simulink model "Regler_08"  (R2014b)
settings: Solver=ode45  StartTime=0.0  StopTime=10.0  RelTol=1e-3
values from neighbouring files (symbols this model uses):
  parInit =     [parameter_08.mat]
  parSys =     [parameter_08.mat]
settings Model: CovSFcnEnable=on  Creator=cds-lue-1  LastModifiedBy=cds-lue-1
settings DebuggingCC: SolverPrmCheckMsg=none  FrameProcessingCompatibilityMsg=error

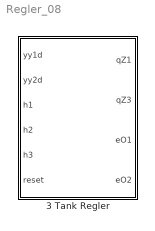
== system Regler_08 ==
  3 Tank Regler : MATLAB Function  TreatAsAtomicUnit=on
      settings: PermitHierarchicalResolution=ParametersOnly

== matlab function Regler_08/3 Tank Regler ==
  settings: updateMethod=DISCRETE  sampleTime=parSys.Ta
  data: qZ1 output; qZ3 output; yy1d input; yy2d input; h1 input; h2 input; h3 input; reset input; parSys parameter; parInit parameter; eO1 output; eO2 output
function [qZ1,qZ3,eO1,eO2]  = fcn(yy1d, yy2d, h1, h2, h3, reset, parSys, parInit)

persistent e1
persistent e2

if isempty(e1)
    e1 = 0;
end

if isempty(e2)
    e2 = 0;
end

if reset
    e1 = 0;
    e2 = 0;
end
    

Atank = parSys.Atank;
rho = parSys.rho;
eta = parSys.eta;
g = parSys.g;
alphaA1 = parSys.alphaA1;
DA1 = parSys.DA1;
alphaA2 = parSys.alphaA2;
A2 = parSys.A2;
alphaA3 = parSys.alphaA3;
DA3 = parSys.DA3;
alpha12_0 = parSys.alpha12_0;
A12 = parSys.A12;
Dh12 = parSys.Dh12;
lambdac12 = parSys.lambdac12;
alpha23_0 = parSys.alpha23_0;
D23 = parSys.D23;
lambdac23 = parSys.lambdac23;
hmin = parSys.hmin;
hmax = parSys.hmax;
dh12min = parSys.dh12min;
a0 = parInit.a0;
a1 = parInit.a1;
dh23min = parSys.dh12min;

A3 = DA3^2*pi/4;
%laut angabe
Dh23 = D23;
A23 = D23^2*pi/4;

y1dpp = yy1d(3);
y1dp  = yy1d(2);
y1d   = yy1d(1);

y2dp  = yy2d(2);
y2d   = yy2d(1);


qA1 = alphaA1 * DA1 ^ 2 * pi * sqrt(0.2e1) * sqrt(g) * sqrt(h1) / 0.4e1;
qA2 = alphaA2 * A2 * sqrt(0.2e1) * sqrt(g) * sqrt(h2);
qA3 = alphaA3 * DA3 ^ 2 * pi * sqrt(0.2e1) * sqrt(g) * sqrt(h3) / 0.4e1;


dqA2_dh2 = alphaA2 * A2 * sqrt(0.2e1) * sqrt(g) * h2 ^ (-0.1e1 / 0.2e1) / 0.2e1;

if abs(h1-h2) > dh12min
    dq12_dh1 = 0.2e1 * alpha12_0 * Dh12 * rho / eta * g / lambdac12 * (0.1e1 - tanh(0.2e1 * Dh12 * rho / eta * sqrt(0.2e1) * sqrt(g) * sqrt(abs(h1 - h2)) / lambdac12) ^ 2) * A12 + alpha12_0 * tanh(0.2e1 * Dh12 * rho / eta * sqrt(0.2e1) * sqrt(g) * sqrt(abs(h1 - h2)) / lambdac12) * A12 * sqrt(0.2e1) * sqrt(g) * (abs(h1 - h2) ^ (-0.1e1 / 0.2e1)) / 0.2e1;
    dq12_dh2 = -0.2e1 * alpha12_0 * Dh12 * rho / eta * g / lambdac12 * (0.1e1 - tanh(0.2e1 * Dh12 * rho / eta * sqrt(0.2e1) * sqrt(g) * sqrt(abs(h1 - h2)) / lambdac12) ^ 2) * A12 - alpha12_0 * tanh(0.2e1 * Dh12 * rho / eta * sqrt(0.2e1) * sqrt(g) * sqrt(abs(h1 - h2)) / lambdac12) * A12 * sqrt(0.2e1) * sqrt(g) * (abs(h1 - h2) ^ (-0.1e1 / 0.2e1)) / 0.2e1;
else
    %Linearisierung
    dq12_dh1 = parSys.d_dq12_dh1 + parSys.k_dq12_dh1*abs(h1-h2);
    dq12_dh2 = parSys.d_dq12_dh2 + parSys.k_dq12_dh2*abs(h1-h2);
end

if abs(h2-h3) > dh23min
    dq23_dh2 = alpha23_0 * D23 ^ 3 * rho / eta * g / lambdac23 * (0.1e1 - tanh(0.2e1 * D23 * rho / eta * sqrt(0.2e1) * sqrt(g) * sqrt(abs(h2 - h3)) / lambdac23) ^ 2) * pi / 0.2e1 + alpha23_0 * tanh(0.2e1 * D23 * rho / eta * sqrt(0.2e1) * sqrt(g) * sqrt(abs(h2 - h3)) / lambdac23) * D23 ^ 2 * pi * sqrt(0.2e1) * sqrt(g) * (abs(h2 - h3) ^ (-0.1e1 / 0.2e1)) / 0.8e1;
    dq23_dh3 = -alpha23_0 * D23 ^ 3 * rho / eta * g / lambdac23 * (0.1e1 - tanh(0.2e1 * D23 * rho / eta * sqrt(0.2e1) * sqrt(g) * sqrt(abs(h2 - h3)) / lambdac23) ^ 2) * pi / 0.2e1 - alpha23_0 * tanh(0.2e1 * D23 * rho / eta * sqrt(0.2e1) * sqrt(g) * sqrt(abs(h2 - h3)) / lambdac23) * D23 ^ 2 * pi * sqrt(0.2e1) * sqrt(g) * (abs(h2 - h3) ^ (-0.1e1 / 0.2e1)) / 0.8e1;
else
    %Linearisierung
    dq23_dh2 = parSys.d_dq23_dh2 + parSys.k_dq23_dh2*abs(h2-h3);
    dq23_dh3 = parSys.d_dq23_dh3 + parSys.k_dq23_dh3*abs(h2-h3);
end

q12 = alpha12_0 * tanh(0.2e1 * Dh12 * rho / eta * sqrt(0.2e1) * sqrt(g) * sqrt(abs(h1 - h2)) / lambdac12) * A12 * sqrt(0.2e1) * sqrt(g) * sqrt(abs(h1 - h2)) * sign((h1 - h2));
q23 = alpha23_0 * tanh(0.2e1 * D23 * rho / eta * sqrt(0.2e1) * sqrt(g) * sqrt(abs(h2 - h3)) / lambdac23) * D23 ^ 2 * pi * sqrt(0.2e1) * sqrt(g) * sqrt(abs(h2 - h3)) * sign((h2 - h3)) / 0.4e1;

Lf1h1 = (q12 - q23 - qA2) / Atank;
Lf2h1 = dq12_dh1 / Atank ^ 2 * (-q12 - qA1) + (dq12_dh2 - dq23_dh2 - dqA2_dh2) / Atank ^ 2 * (q12 - q23 - qA2) - dq23_dh3 / Atank ^ 2 * (q23 - qA3);
Lg1Lf1h1 = dq12_dh1 / Atank ^ 2;
Lg2Lf1h1 = -dq23_dh3 / Atank ^ 2;
Lg1h2 = 0.1e1 / Atank;
Lg2h2 = -0.1e1 / Atank;
Lf1h2 = (-q12 - qA1) / Atank - (q23 - qA3) / Atank;

% v um I-Anteil schon erweitert
v = [y1dpp - parInit.a10 * (h2 - y1d) - parInit.a11 * (Lf1h1 - y1dp) - parInit.a1I * e1;
     y2dp  - parInit.a20 * (h1 - h3 - y2d) - parInit.a2I * e2
     ];

bb = [Lf2h1; Lf1h2;];
DD_inv = [-Lg2h2 / (Lg1h2 * Lg2Lf1h1 - Lg2h2 * Lg1Lf1h1) Lg2Lf1h1 / (Lg1h2 * Lg2Lf1h1 - Lg2h2 * Lg1Lf1h1); Lg1h2 / (Lg1h2 * Lg2Lf1h1 - Lg2h2 * Lg1Lf1h1) -Lg1Lf1h1 / (Lg1h2 * Lg2Lf1h1 - Lg2h2 * Lg1Lf1h1);];
u_temp = DD_inv*(-bb+v);
qZ1 = u_temp(1);
qZ3 = u_temp(2);

%Anti-Windup
if qZ1 < parSys.qZ1max && qZ1 > parSys.qZ1min && qZ3 < parSys.qZ3max && qZ3 > parSys.qZ3min
    e1 = e1 + (h2 - y1d)*parSys.Ta;
    e2 = e2 + (h1 - h3 - y2d)*parSys.Ta;
end

eO1 = e1;
eO2 = e2;

end
